simulink subsystem "subrUnwrap"  (R2024a)
settings: Solver=VariableStepAuto  StartTime=0.0  StopTime=10.0  RelTol=1e-3
settings Model: Creator=anant  LastModifiedBy=anant

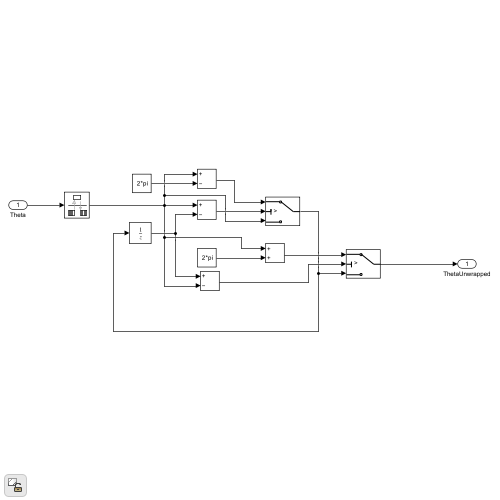
[thumbnail: Simulink's stored preview of the top-level diagram]
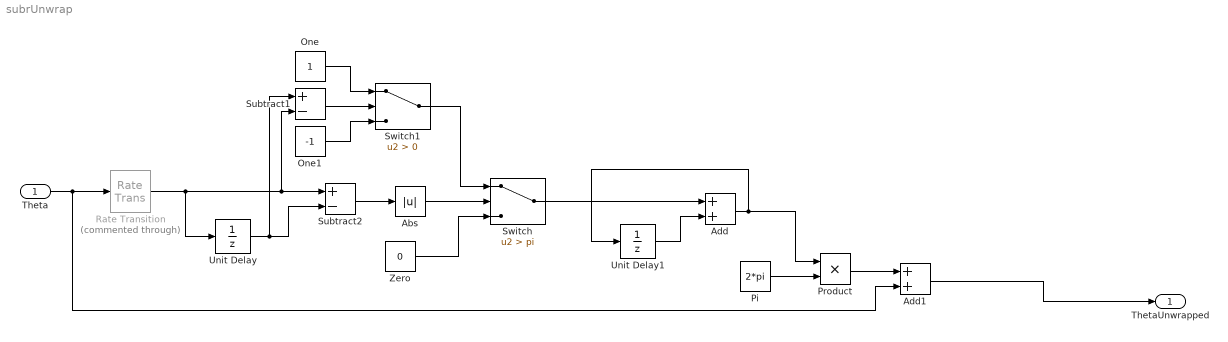
== system subrUnwrap ==
  Theta : Inport
  Abs : Abs  SaturateOnIntegerOverflow=off
  Add : Sum
  Add1 : Sum
  One : Constant  OutDataTypeStr=Inherit: Inherit via back propagation
  One1 : Constant  Value=-1  OutDataTypeStr=Inherit: Inherit via back propagation
  Pi : Constant  Value=2*pi  OutDataTypeStr=Inherit: Inherit via back propagation
  Product : Product
  Rate Transition : RateTransition  Commented=through
  Subtract1 : Sum  Inputs=+-
  Subtract2 : Sum  Inputs=+-
  Switch : Switch  Criteria=u2 > Threshold  Threshold=pi  SaturateOnIntegerOverflow=off  InputSameDT=off
  Switch1 : Switch  Criteria=u2 > Threshold  SaturateOnIntegerOverflow=off  InputSameDT=off
  Unit Delay : UnitDelay  SampleTime=-1  HasFrameUpgradeWarning=on
  Unit Delay1 : UnitDelay  SampleTime=-1  HasFrameUpgradeWarning=on
  Zero : Constant  Value=0  OutDataTypeStr=Inherit: Inherit via back propagation
  ThetaUnwrapped : Outport
  wires:
  Rate Transition/1 -> Subtract2/1, Subtract1/2, Unit Delay/1
  Unit Delay/1 -> Subtract2/2, Subtract1/1
  Add1/1 -> ThetaUnwrapped/1
  Subtract2/1 -> Abs/1
  Zero/1 -> Switch/3
  Abs/1 -> Switch/2
  Subtract1/1 -> Switch1/2
  One/1 -> Switch1/1
  One1/1 -> Switch1/3
  Switch1/1 -> Switch/1
  Switch/1 -> Add/1
  Add/1 -> Unit Delay1/1, Product/1
  Unit Delay1/1 -> Add/2
  Pi/1 -> Product/2
  Product/1 -> Add1/1
  Theta/1 -> Rate Transition/1, Add1/2
